simulink model "part2_project_file"  (R2023b)
settings: Solver=VariableStepAuto  StartTime=0.0  StopTime=30  RelTol=1e-3
values from neighbouring files (symbols this model uses):
  air_density = 1.225    [post_credit_scene.m]    (also in simulink_part2B_link.m; simulink_part2_link.m)
  alpha_n = alpha_n_array(i)    [post_credit_scene.m]    (also in simulink_part2B_link.m = 16; simulink_part2_link.m = alpha_n_array(5))
  area = 2.4    [post_credit_scene.m]    (also in simulink_part2B_link.m; simulink_part2_link.m)
  beta = 0.4    [post_credit_scene.m]    (also in simulink_part2B_link.m; simulink_part2_link.m)
  drag_coefficient = 0.32    [post_credit_scene.m]    (also in simulink_part2B_link.m; simulink_part2_link.m)
  gradient = 0    [post_credit_scene.m]    (also in simulink_link.m; simulink_part2_link.m = deg2rad(0))
  gravity = 9.81    [post_credit_scene.m]    (also in simulink_part2B_link.m; simulink_part2_link.m)
  initial_speed = 0    [post_credit_scene.m]    (also in simulink_link.m; simulink_part2B_link.m; simulink_part2_link.m)
  Ki_m2 = 0.1    [post_credit_scene.m]    (also in simulink_part2B_link.m; simulink_part2_link.m)
  Kp_m2 = 0.5    [post_credit_scene.m]    (also in simulink_part2B_link.m; simulink_part2_link.m)
  linear_slope = (26.82) / zero_to_sixty    (= 3.08275862069)    [post_credit_scene.m]    (also in simulink_link.m = 3.44827586207; simulink_part2_link.m = 3.44827586207)
  mass = 1000    [post_credit_scene.m]    (also in simulink_part2B_link.m; simulink_part2_link.m)
  max_engine_revs = 420    [post_credit_scene.m]    (also in simulink_part2B_link.m; simulink_part2_link.m)
  max_speed = 30    [post_credit_scene.m]    (also in simulink_link.m; simulink_part2B_link.m = 60; simulink_part2_link.m)
  max_torque = 190    [post_credit_scene.m]    (also in simulink_part2B_link.m; simulink_part2_link.m)
  rolling_coefficient = 0.01    [post_credit_scene.m]    (also in simulink_part2B_link.m; simulink_part2_link.m)
libraries: simulink x1
settings Model: PacingRate=0.001300  Creator=Matthew  LastModifiedBy=Matthew

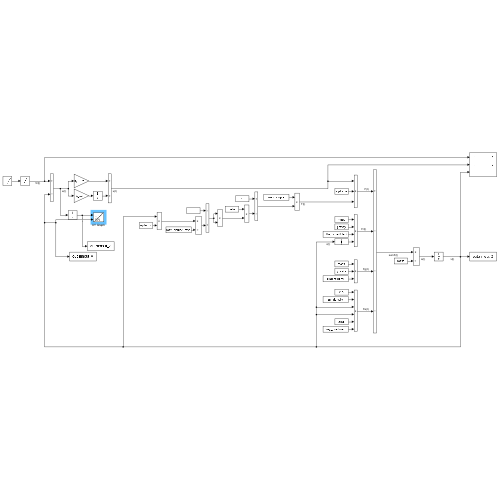
[thumbnail: Simulink's stored preview of the top-level diagram]
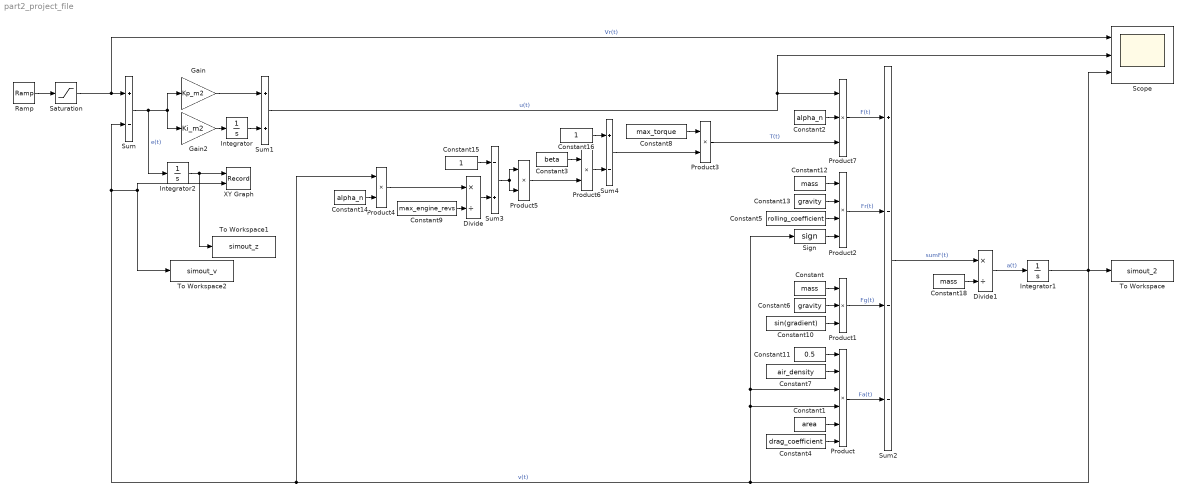
== system part2_project_file ==
  Constant : Constant  Value=mass
  Constant1 : Constant  Value=area
  Constant10 : Constant  Value=sin(gradient)
  Constant11 : Constant  Value=0.5
  Constant12 : Constant  Value=mass
  Constant13 : Constant  Value=gravity
  Constant14 : Constant  Value=alpha_n
  Constant15 : Constant
  Constant16 : Constant
  Constant18 : Constant  Value=mass
  Constant2 : Constant  Value=alpha_n
  Constant3 : Constant  Value=beta
  Constant4 : Constant  Value=drag_coefficient
  Constant5 : Constant  Value=rolling_coefficient
  Constant6 : Constant  Value=gravity
  Constant7 : Constant  Value=air_density
  Constant8 : Constant  Value=max_torque
  Constant9 : Constant  Value=max_engine_revs
  Divide : Product  Inputs=*/
  Divide1 : Product  Inputs=*/
  Gain : Gain  Gain=Kp_m2
  Gain2 : Gain  Gain=Ki_m2
  Integrator : Integrator
  Integrator1 : Integrator
  Integrator2 : Integrator
  Product : Product  Inputs=6
  Product1 : Product  Inputs=3
  Product2 : Product  Inputs=4
  Product{3..6} (4 alike) : Product
  Product7 : Product  Inputs=3
  Ramp : simulink/Sources/Ramp  slope=linear_slope  start=0  InitialOutput=0
  Saturation : Saturate  UpperLimit=max_speed  LowerLimit=initial_speed
  Scope : Scope  NumInputPorts=3
  Sign : Signum
  Sum : Sum  Inputs=+-
  Sum1 : Sum
  Sum2 : Sum  Inputs=+---
  Sum3 : Sum  Inputs=-+
  Sum4 : Sum  Inputs=+-
  To Workspace : ToWorkspace  VariableName=simout_2  SaveFormat=Timeseries  SampleTime=-1
  To Workspace1 : ToWorkspace  VariableName=simout_z  SaveFormat=Timeseries  SampleTime=-1
  To Workspace2 : ToWorkspace  VariableName=simout_v  SaveFormat=Timeseries  SampleTime=-1
  XY Graph : Record  VariableName=z_v_phaseplot  RecordToWorkspace=on  FileSettingsInternal="{\"entries\":[{\"content\":{\"excelSettings\":{\"content\":{},\"type\":\"Streamout.ExcelSettings\"}},\"type\":\"Streamout.FileSettingStorage\",\"uuid\":\"\"}],\"packageUris\":[\"http:\\/\\/schema.mathworks.com\\/mf0\\/streamout_blocks\\/R2020a\"],\"version\":\"1.0\"}"  Layout=[1 1]  SignalsInternal="{\"entries\":[{\"content\":{\"signals\":[{\"content\":{\"blockPath\":[],\"dimensions\":[1],\"domain\":\"\",\"lineColor\":\"#a2142f\",\"plots\":[1],\"port\":1,\"sid\":[\"\"],\"signalID\":625,\"signalName\":\"Integrator2\"},\"type\":\"RecordBlkView.Signal\",\"uuid\":\"\"},{\"content\":{\"blockPath\":[],\"dimensions\":[1],\"domain\":\"\",\"lineColor\":\"#139fff\",\"plots\":[1],\"port\":2,\"sid\":[\"\"],\"signalID\":629,\"signalName\":\"v(t)\"},\"type\":\"RecordBlkView.Signal\",\"uuid\":\"\"}]},\"type\":\"RecordBlkView.InputSignals\",\"uuid\":\"\"}],\"packageUris\":[\"http:\\/\\/schema.mathworks.com\\/mf0\\/streamout_blocks\\/R2020a\"],\"version\":\"1.0\"}"  VisualizationBindings="{\"xyplotplugin\":{\"info\":[{\"series\":[{\"bindingParametersList\":[{\"parameter\":\"X-Axis\",\"signalID\":625,\"signalName\":\"Integrator2\"},{\"parameter\":\"Y-Axis\",\"signalID\":629,\"signalName\":\"v(t)\"}],\"seriesID\":23604}],\"subplotID\":1}]}}"  CompatibilityTag=XY
  wires:
  Ramp/1 -> Saturation/1
  Saturation/1 -> Scope/1, Sum/1  "Vr(t)"
  Sum/1 -> Integrator2/1, Gain/1, Gain2/1  "e(t)"
  Gain2/1 -> Integrator/1
  Integrator/1 -> Sum1/2
  Gain/1 -> Sum1/1
  Constant11/1 -> Product/1
  Constant4/1 -> Product/6
  Constant7/1 -> Product/2
  Constant1/1 -> Product/5
  Product/1 -> Sum2/4  "Fa(t)"
  Constant/1 -> Product1/1
  Constant6/1 -> Product1/2
  Constant10/1 -> Product1/3
  Product1/1 -> Sum2/3  "Fg(t)"
  Product2/1 -> Sum2/2  "Fr(t)"
  Constant5/1 -> Product2/3
  Constant12/1 -> Product2/1
  Constant13/1 -> Product2/2
  Sign/1 -> Product2/4
  Divide1/1 -> Integrator1/1  "a(t)"
  Constant9/1 -> Divide/2
  Product4/1 -> Divide/1
  Constant8/1 -> Product3/1
  Constant14/1 -> Product4/2
  Constant15/1 -> Sum3/1
  Divide/1 -> Sum3/2
  Sum3/1 -> Product5/2, Product5/1
  Constant3/1 -> Product6/1
  Product5/1 -> Product6/2
  Product6/1 -> Sum4/2
  Constant16/1 -> Sum4/1
  Sum4/1 -> Product3/2
  Constant2/1 -> Product7/2
  Product7/1 -> Sum2/1  "F(t)"
  Sum2/1 -> Divide1/1  "sumF(t)"
  Constant18/1 -> Divide1/2
  Integrator1/1 -> To Workspace/1, Scope/3, Sign/1, Product/3, Product/4, Product4/1, Sum/2, XY Graph/2, To Workspace2/1  "v(t)"
  Product3/1 -> Product7/3  "T(t)"
  Sum1/1 -> Scope/2, Product7/1  "u(t)"
  Integrator2/1 -> To Workspace1/1, XY Graph/1
